simulink model "hw8"  (R2019a)
settings: Solver=VariableStepAuto  StartTime=0  StopTime=260  RelTol=1e-3
undefined symbols (not defined in the file): DiscIntNeverNeededParam
settings Model: Creator=sumli  LastModifiedBy=sumli

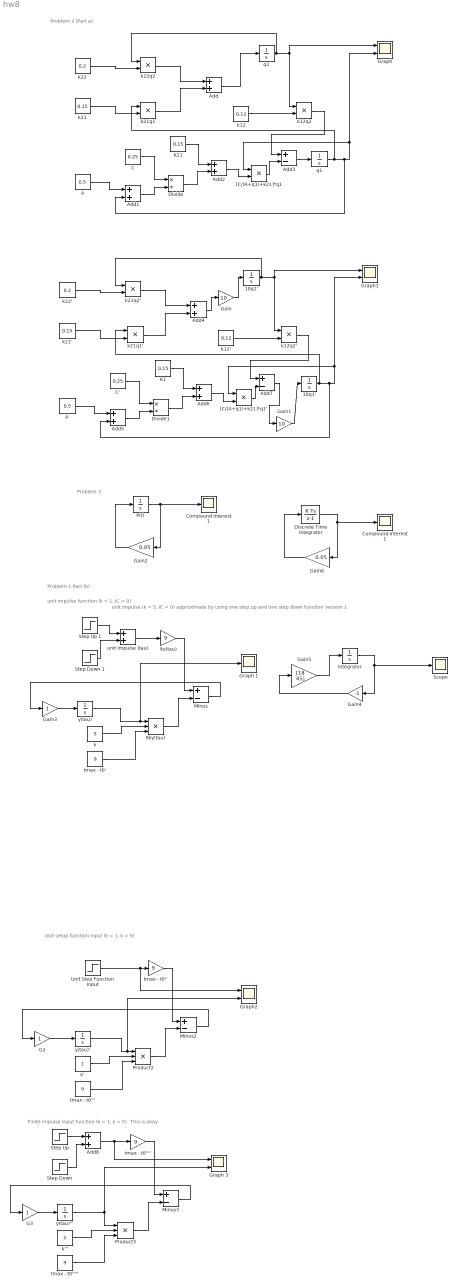
== system hw8 ==
  note: This is okay
  note: Finite impulse input function (k = 1, k = 5)
  note: Unit setup function input (k = 1, k = 5)
  note: version 1
  note: approximate by using one step up and one step down function
  note: unit impulse (k = 5, IC = 0)
  note: unit impulse function (k = 1, IC = 0)
  note: Problem 3
  note: Problem 1 Part (b)
  note: Problem 2 (Part a)
  10q1' : Integrator  InitialCondition=100
  10q2' : Integrator  InitialCondition=100
  9ky(tau) : Product  Inputs=3
  9u(tau) : Gain  Gain=9
  A : Constant  Value=0.5
  A' : Constant  Value=0.5
  Add{,1..2,4..6,8} (7 alike) : Sum
  Add3 : Sum  Inputs=+-
  Add7 : Sum  Inputs=+-
  C : Constant  Value=0.25
  C' : Constant  Value=0.25
  Compound Interest 1 : Scope
  "Compound Interest 1 " : Scope
  Discrete Time Integrator : DiscreteIntegrator  InitialCondition=1000  SampleTime=-1  ICPrevOutput=DiscIntNeverNeededParam  ICPrevScaledInput=DiscIntNeverNeededParam
  Divide : Product  Inputs=*/
  Divide1 : Product  Inputs=*/
  G2 : Gain
  G3 : Gain
  Gain : Gain  Gain=10
  Gain1 : Gain  Gain=10
  Gain2 : Gain  Gain=0.05
  Gain3 : Gain
  Gain4 : Gain  Gain=-1
  Gain5 : Gain  Gain=[18 45]
  Gain6 : Gain  Gain=0.05
  Graph : Scope  NumInputPorts=2
  Graph 1 : Scope
  Graph 3 : Scope  NumInputPorts=2
  Graph1 : Scope  NumInputPorts=2
  Graph2 : Scope  NumInputPorts=2
  Integrator : Integrator  InitialCondition=1
  K1 : Constant  Value=0.15
  K21 : Constant  Value=0.15
  Minus : Sum  Inputs=+-
  Minus2 : Sum  Inputs=+-
  Minus3 : Sum  Inputs=+-
  P(t) : Integrator  InitialCondition=1000
  Product2 : Product  Inputs=3
  Product3 : Product  Inputs=3
  Scope : Scope
  Step Down : Step  Time=1/9  After=-1  SampleTime=0
  "Step Down 1 " : Step  Time=0.000001  After=-1000000  SampleTime=0
  Step Up : Step  Time=0  SampleTime=0
  Step Up 1 : Step  Time=0  After=1000000  SampleTime=0
  "Unit Step Function Input " : Step  SampleTime=0
  "[C/(A+q1)+k21]*q1" : Product
  "[C/(A+q1)+k21]*q1'" : Product
  k : Constant  Value=5
  k' : Constant
  k''' : Constant  Value=5
  k12 : Constant  Value=0.12
  k12' : Constant  Value=0.12
  k12q2 : Product
  k12q2' : Product
  k21 : Constant  Value=0.15
  k21' : Constant  Value=0.15
  k21q1 : Product
  k21q1' : Product
  k22 : Constant  Value=0.2
  k22' : Constant  Value=0.2
  k22q2 : Product
  k22q2' : Product
  q1 : Integrator  InitialCondition=100
  q2 : Integrator  InitialCondition=100
  tmax - t0' : Constant  Value=9
  tmax - t0'' : Gain  Gain=9
  tmax - t0''' : Constant  Value=9
  tmax - t0'''' : Gain  Gain=9
  tmax - t0''''' : Constant  Value=9
  unit impulse (tau) : Sum
  y(tau) : Integrator
  y(tau)' : Integrator
  y(tau)''' : Integrator
  wires:
  k22q2/1 -> Add/1
  k21q1/1 -> Add/2
  k22/1 -> k22q2/2
  k21/1 -> k21q1/2
  Add/1 -> q2/1
  q2/1 -> k22q2/1, k12q2/1, Graph/1
  k12/1 -> k12q2/2
  A/1 -> Add1/1
  C/1 -> Divide/1
  K21/1 -> Add2/1
  Add1/1 -> Divide/2
  Divide/1 -> Add2/2
  Add2/1 -> "[C/(A+q1)+k21]*q1"/2
  "[C/(A+q1)+k21]*q1"/1 -> Add3/2
  k12q2/1 -> Add3/1
  q1/1 -> k21q1/1, Add1/2, "[C/(A+q1)+k21]*q1"/1, Graph/2
  Add3/1 -> q1/1
  A'/1 -> Add5/1
  k22q2'/1 -> Add4/1
  Add5/1 -> Divide1/2
  k22'/1 -> k22q2'/2
  "[C/(A+q1)+k21]*q1'"/1 -> Add7/2
  C'/1 -> Divide1/1
  Add6/1 -> "[C/(A+q1)+k21]*q1'"/2
  k21'/1 -> k21q1'/2
  K1/1 -> Add6/1
  10q2'/1 -> k22q2'/1, k12q2'/1, Graph1/1
  k21q1'/1 -> Add4/2
  k12q2'/1 -> Add7/1
  k12'/1 -> k12q2'/2
  Divide1/1 -> Add6/2
  10q1'/1 -> k21q1'/1, Add5/2, "[C/(A+q1)+k21]*q1'"/1, Graph1/2
  Add4/1 -> Gain/1
  Gain/1 -> 10q2'/1
  Add7/1 -> Gain1/1
  Gain1/1 -> 10q1'/1
  P(t)/1 -> Gain2/1, "Compound Interest 1 "/1
  Gain2/1 -> P(t)/1
  Step Up 1/1 -> unit impulse (tau)/1
  "Step Down 1 "/1 -> unit impulse (tau)/2
  unit impulse (tau)/1 -> 9u(tau)/1
  k/1 -> 9ky(tau)/2
  tmax - t0'/1 -> 9ky(tau)/3
  9u(tau)/1 -> Minus/1
  9ky(tau)/1 -> Minus/2
  tmax - t0''/1 -> Minus2/1
  k'/1 -> Product2/2
  Product2/1 -> Minus2/2
  tmax - t0'''/1 -> Product2/3
  y(tau)'/1 -> Graph2/2, Product2/1
  "Unit Step Function Input "/1 -> Graph2/1, tmax - t0''/1
  tmax - t0''''/1 -> Minus3/1
  y(tau)'''/1 -> Graph 3/2, Product3/1
  Product3/1 -> Minus3/2
  k'''/1 -> Product3/2
  tmax - t0'''''/1 -> Product3/3
  Add8/1 -> Graph 3/1, tmax - t0''''/1
  Step Up/1 -> Add8/1
  Step Down/1 -> Add8/2
  y(tau)/1 -> Graph 1/1, 9ky(tau)/1
  G2/1 -> y(tau)'/1
  Minus2/1 -> G2/1
  G3/1 -> y(tau)'''/1
  Minus3/1 -> G3/1
  Integrator/1 -> Scope/1, Gain4/1
  Gain4/1 -> Gain5/1
  Gain5/1 -> Integrator/1
  Gain3/1 -> y(tau)/1
  Minus/1 -> Gain3/1
  Gain6/1 -> Discrete Time Integrator/1
  Discrete Time Integrator/1 -> Gain6/1, Compound Interest 1/1
